simulink model "Three Phase SPWM"  (R2017a)
settings: Solver=ode45  StartTime=0.0  StopTime=0.1  MaxStep=1e-6  RelTol=1e-3  EnableMultiTasking=on
libraries: powerlib x15, powerlib_extras x3, simulink x1
settings Model: Creator=Kashif  LastModifiedBy=sujee
settings DataIOCC: LimitDataPoints=on  SaveFormat=Array  SignalLoggingSaveFormat=ModelDataLogs
settings OptimizationCC: ExpressionDepthLimit=2147483647  LifeSpan=inf
settings DebuggingCC: UnderspecifiedInitializationDetection=Classic  MergeDetectMultiDrivingBlocksExec=none  SolverPrmCheckMsg=warning  FcnCallInpInsideContextMsg=warning  StateNameClashWarn=warning  SFUnexpectedBacktrackingDiag=warning  SFNoUnconditionalDefaultTransitionDiag=warning  SFExecutionAtInitializationDiag=none
settings HardwareCC: ProdBitPerPointer=32  ProdBitPerSizeT=32  ProdBitPerPtrDiffT=32  ProdLargestAtomicFloat=None  ProdIntDivRoundTo=Undefined  ProdEndianess=Unspecified  ProdWordSize=32  ProdHWDeviceType=32-bit Generic
settings ModelReferenceCC: PropagateSignalLabelsOutOfModel=off
settings GRTTargetCC: TargetLangStandard=C89/C90 (ANSI)  CombineOutputUpdateFcns=off  GRTInterface=on
settings ConfigComp: CovMetricSettings=dw  CovSaveCumulativeToWorkspaceVar=on  CovSaveSingleToWorkspaceVar=on  CovExternalEMLEnable=off
settings SimscapeCC: SimscapeNormalizeSystem=off

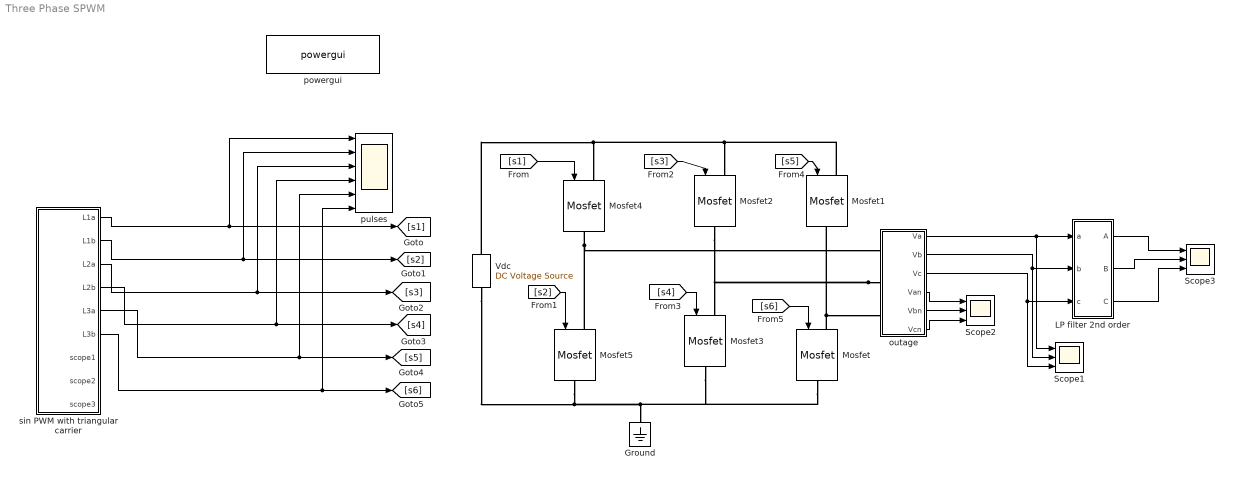
== system Three Phase SPWM ==
  Ground : powerlib/Elements/Ground  LConnTagsString=a
  LP filter 2nd order : Subsystem  mask{cutoff_frequency=200, damping_factor=0.707}
      mask prompts: cutoff_frequency "Cut off frequency"; damping_factor "Damping Factor"
  Mosfet{,1..5} (6 alike) : powerlib/Power Electronics/Mosfet  Ron=0.1  Lon=0  Rd=0.01  Vfd=0  IC=0  Rs=1e5  Cs=inf  Measurements=off
  Scope1 : Scope  NumInputPorts=3
  Scope2 : Scope  NumInputPorts=3
  Scope3 : Scope  NumInputPorts=3
  Vdc : powerlib/Electrical Sources/DC Voltage Source  Amplitude=400  Measurements=None
  outage : Subsystem
  powergui : powerlib/powergui  Priority=1  SimulationMode=Discrete  SampleTime=2e-6  frequency=60  Iterations=50  frequencyindice=0  Pbase=100e6  ErrMax=1e-4  UnitsV=kV  UnitsW=MW  buscounter=0  FunctionMessages=off  echomessages=off  EnableUseOfTLC=off  CurrentSourceSwitches=off  DisableSnubberDevices=off  DisableRonSwitches=off  DisableVfSwitches=off  DisplayEquations=off  AutomaticDiscreteSolvers=off  SolverType=Tustin/Backward Euler (TBE)  Interpol=off  ExternalGateDelay=off  methode=off  Ts=0  x0status=blocks  SPID=off  SwTol=0  HookPort=off  NonlinearTolerance=1e-4  nMaxIteration=100  ContinueOnMaxIteration=off  RestoreLinks=warning  ResistiveCurrentMeasurement=off  Frange=[0:2:500]  Ylog=off  Xlog=on  ShowGrid=off  save=off  variable=ZData  structure=Line_voltages  ZoomFFT=off  StartTime=0.04  cycles=1  DisplayStyle=2  fundamental=50  FreqAxis=off  MaxFrequency=10000  frequencyindicesteady=1  RmsSteady=1  display=off
  pulses : Scope  NumInputPorts=6
  sin PWM with triangular carrier : Subsystem  mask{mi=10, freq=50, fs=2000}
      mask prompts: mi "mi(0 to 1)"; freq "Output frequency"; fs "Switching frequency"
  wires:
  [s1] -> Mosfet4/1
  sin PWM with triangular carrier/2(L1b) -> [s2], pulses/2
  [s2] -> Mosfet5/1
  [s3] -> Mosfet2/1
  sin PWM with triangular carrier/3(L2a) -> pulses/3, [s3]
  [s4] -> Mosfet3/1
  sin PWM with triangular carrier/4(L2b) -> [s4], pulses/4
  [s5] -> Mosfet1/1
  [s6] -> Mosfet/1
  sin PWM with triangular carrier/6(L3b) -> [s6], pulses/6
  outage/1(Va) -> Scope1/1, LP filter 2nd order/1(a)
  outage/2(Vb) -> Scope1/2, LP filter 2nd order/2(b)
  outage/3(Vc) -> Scope1/3, LP filter 2nd order/3(c)
  sin PWM with triangular carrier/1(L1a) -> pulses/1, [s1]
  sin PWM with triangular carrier/5(L3a) -> [s5], pulses/5
  outage/4(Van) -> Scope2/1
  outage/5(Vbn) -> Scope2/2
  outage/6(Vcn) -> Scope2/3
  LP filter 2nd order/1(A) -> Scope3/1
  LP filter 2nd order/2(B) -> Scope3/2
  LP filter 2nd order/3(C) -> Scope3/3
  connections:
  Mosfet1/LConn1 -- Mosfet2/LConn1 -- Mosfet4/LConn1 -- Vdc/RConn1
  Mosfet4/RConn1 -- Mosfet5/LConn1 -- outage/LConn1
  Mosfet/LConn1 -- Mosfet1/RConn1 -- outage/LConn3
  Vdc/LConn1 -- Mosfet5/RConn1 -- Mosfet/RConn1 -- Mosfet3/RConn1 -- Ground/LConn1
  outage/LConn2 -- Mosfet2/RConn1 -- Mosfet3/LConn1

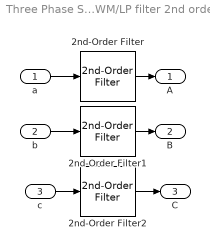
== system Three Phase SPWM/LP filter 2nd order ==
  a : Inport
  b : Inport  Port=2
  c : Inport  Port=3
  2nd-Order Filter : powerlib_extras/Control  Blocks/2nd-Order Filter  FilterType=Lowpass  Fo=cutoff_frequency  Zeta=damping_factor  Initialize=off  Vac_Init=[1 45 60]  Vdc_Init=-0.5  PlotResponse=off  param1=[1 500 1]
      settings: SourceProductBaseCode=PS
  2nd-Order Filter1 : powerlib_extras/Control  Blocks/2nd-Order Filter  FilterType=Lowpass  Fo=cutoff_frequency  Zeta=damping_factor  Initialize=off  Vac_Init=[1 45 60]  Vdc_Init=-0.5  PlotResponse=off  param1=[1 500 1]
      settings: SourceProductBaseCode=PS
  2nd-Order Filter2 : powerlib_extras/Control  Blocks/2nd-Order Filter  FilterType=Lowpass  Fo=cutoff_frequency  Zeta=damping_factor  Initialize=off  Vac_Init=[1 45 60]  Vdc_Init=-0.5  PlotResponse=off  param1=[1 500 1]
      settings: SourceProductBaseCode=PS
  A : Outport
  B : Outport  Port=2
  C : Outport  Port=3
  wires:
  a/1 -> 2nd-Order Filter/1
  2nd-Order Filter/1 -> A/1
  b/1 -> 2nd-Order Filter1/1
  2nd-Order Filter1/1 -> B/1
  c/1 -> 2nd-Order Filter2/1
  2nd-Order Filter2/1 -> C/1

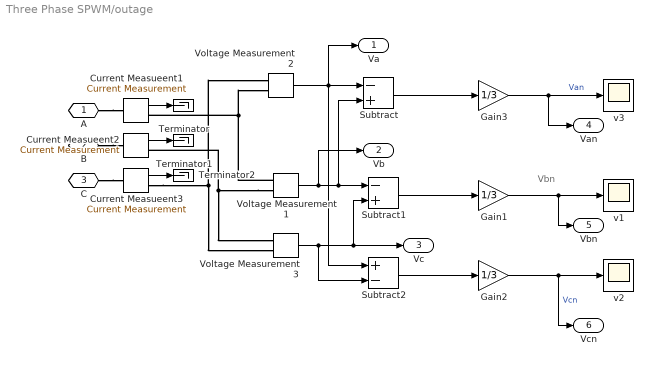
== system Three Phase SPWM/outage ==
  note: Vbn
  Current Measueent1 : powerlib/Measurements/Current Measurement  PhasorSimulation=off  OutputType=Complex  PSBequivalent=0
  Current Measueent2 : powerlib/Measurements/Current Measurement  PhasorSimulation=off  OutputType=Complex  PSBequivalent=0
  Current Measueent3 : powerlib/Measurements/Current Measurement  PhasorSimulation=off  OutputType=Complex  PSBequivalent=0
  Gain1 : Gain  Gain=1/3
  Gain2 : Gain  Gain=1/3
  Gain3 : Gain  Gain=1/3
  Subtract : Sum  Inputs=-+
  Subtract1 : Sum  Inputs=-+
  Subtract2 : Sum  Inputs=+-
  Terminator : Terminator
  Terminator1 : Terminator
  Terminator2 : Terminator
  Voltage Measurement1 : powerlib/Measurements/Voltage Measurement  PhasorSimulation=off  OutputType=Complex  PSBequivalent=0
  Voltage Measurement2 : powerlib/Measurements/Voltage Measurement  PhasorSimulation=off  OutputType=Complex  PSBequivalent=0
  Voltage Measurement3 : powerlib/Measurements/Voltage Measurement  PhasorSimulation=off  OutputType=Complex  PSBequivalent=0
  v1 : Scope
  v2 : Scope
  v3 : Scope
  A : PMIOPort  Side=Left
  B : PMIOPort  Port=2  Side=Left
  C : PMIOPort  Port=3  Side=Left
  Va : Outport
  Vb : Outport  Port=2
  Vc : Outport  Port=3
  Van : Outport  Port=4
  Vbn : Outport  Port=5
  Vcn : Outport  Port=6
  wires:
  Gain2/1 -> v2/1, Vcn/1  "Vcn"
  Subtract2/1 -> Gain2/1
  Gain1/1 -> v1/1, Vbn/1
  Subtract1/1 -> Gain1/1
  Voltage Measurement3/1 -> Subtract2/2, Subtract1/2, Vc/1
  Gain3/1 -> v3/1, Van/1  "Van"
  Subtract/1 -> Gain3/1
  Voltage Measurement1/1 -> Subtract/2, Subtract1/1, Vb/1
  Voltage Measurement2/1 -> Subtract/1, Subtract2/1, Va/1
  Current Measueent1/1 -> Terminator/1
  Current Measueent3/1 -> Terminator2/1
  Current Measueent2/1 -> Terminator1/1
  connections:
  Voltage Measurement1/LConn1 -- Current Measueent1/RConn1 -- Voltage Measurement2/LConn2
  Voltage Measurement1/LConn2 -- Current Measueent2/RConn1 -- Voltage Measurement3/LConn1
  Current Measueent3/RConn1 -- Voltage Measurement2/LConn1 -- Voltage Measurement3/LConn2
  A/RConn1 -- Current Measueent1/LConn1
  B/RConn1 -- Current Measueent2/LConn1
  C/RConn1 -- Current Measueent3/LConn1

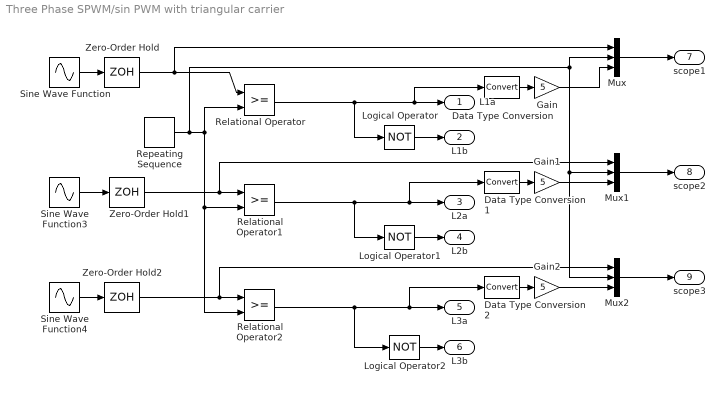
== system Three Phase SPWM/sin PWM with triangular carrier ==
  Data Type Conversion : DataTypeConversion
  Data Type Conversion1 : DataTypeConversion
  Data Type Conversion2 : DataTypeConversion
  Gain : Gain  Gain=5
  Gain1 : Gain  Gain=5
  Gain2 : Gain  Gain=5
  Logical Operator : Logic  Operator=NOT  AllPortsSameDT=off  OutDataTypeStr=boolean
  Logical Operator1 : Logic  Operator=NOT  AllPortsSameDT=off  OutDataTypeStr=boolean
  Logical Operator2 : Logic  Operator=NOT  AllPortsSameDT=off  OutDataTypeStr=boolean
  Mux : Mux  Inputs=3
  Mux1 : Mux  Inputs=3
  Mux2 : Mux  Inputs=3
  Relational Operator : RelationalOperator  OutDataTypeStr=boolean  RndMeth=Nearest
  Relational Operator1 : RelationalOperator  OutDataTypeStr=boolean  RndMeth=Nearest
  Relational Operator2 : RelationalOperator  OutDataTypeStr=boolean  RndMeth=Nearest
  Repeating Sequence : simulink/Sources/Repeating Sequence  rep_seq_t=[0 0.25/fs 0.5/fs 0.75/fs 1/fs]  rep_seq_y=[10 0 -10 0 10]
  Sine Wave Function : Sin  Amplitude=mi  Frequency=freq*2*pi  SampleTime=0
  Sine Wave Function3 : Sin  Amplitude=mi  Frequency=freq*2*pi  Phase=4*pi/3  SampleTime=0
  Sine Wave Function4 : Sin  Amplitude=mi  Frequency=freq*2*pi  Phase=2*pi/3  SampleTime=0
  Zero-Order Hold : ZeroOrderHold  SampleTime=1/fs
  Zero-Order Hold1 : ZeroOrderHold  SampleTime=1/fs
  Zero-Order Hold2 : ZeroOrderHold  SampleTime=1/fs
  L1a : Outport
  L1b : Outport  Port=2
  L2a : Outport  Port=3
  L2b : Outport  Port=4
  L3a : Outport  Port=5
  L3b : Outport  Port=6
  scope1 : Outport  Port=7
  scope2 : Outport  Port=8
  scope3 : Outport  Port=9
  wires:
  Sine Wave Function/1 -> Zero-Order Hold/1
  Repeating Sequence/1 -> Relational Operator/2, Relational Operator1/2, Relational Operator2/2, Mux/2, Mux2/2, Mux1/2
  Relational Operator/1 -> Logical Operator/1, L1a/1, Data Type Conversion/1
  Sine Wave Function3/1 -> Zero-Order Hold1/1
  Sine Wave Function4/1 -> Zero-Order Hold2/1
  Relational Operator1/1 -> Logical Operator1/1, L2a/1, Data Type Conversion1/1
  Relational Operator2/1 -> Logical Operator2/1, L3a/1, Data Type Conversion2/1
  Logical Operator/1 -> L1b/1
  Logical Operator1/1 -> L2b/1
  Logical Operator2/1 -> L3b/1
  Zero-Order Hold/1 -> Relational Operator/1, Mux/1
  Zero-Order Hold1/1 -> Relational Operator1/1, Mux1/1
  Zero-Order Hold2/1 -> Relational Operator2/1, Mux2/1
  Data Type Conversion/1 -> Gain/1
  Gain/1 -> Mux/3
  Gain1/1 -> Mux1/3
  Data Type Conversion1/1 -> Gain1/1
  Data Type Conversion2/1 -> Gain2/1
  Gain2/1 -> Mux2/3
  Mux/1 -> scope1/1
  Mux1/1 -> scope2/1
  Mux2/1 -> scope3/1
